simulink model "problema1_sin_disipador"  (R2017a)
settings: Solver=VariableStepAuto  StartTime=0.0  StopTime=2000  RelTol=1e-3
settings Model: Creator=elsuizo  LastModifiedBy=elsuizo

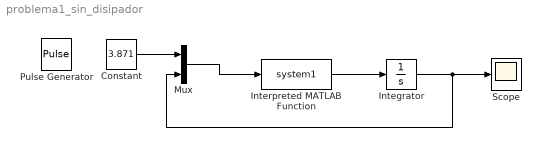
== system problema1_sin_disipador ==
  Constant : Constant  Value=3.871
  Integrator : Integrator
  Interpreted MATLAB Function : MATLABFcn  MATLABFcn=system1  OutputDimensions=2
  Mux : Mux  Inputs=2
  Pulse Generator : DiscretePulseGenerator  PulseType=Time based  Amplitude=175  Period=0.001  PulseWidth=10
  Scope : Scope
  wires:
  Integrator/1 -> Mux/2, Scope/1
  Mux/1 -> Interpreted MATLAB Function/1
  Interpreted MATLAB Function/1 -> Integrator/1
  Constant/1 -> Mux/1
